simulink model "guidance_v1_4_1"  (R2019a)
settings: Solver=FixedStepDiscrete  StartTime=0.0  StopTime=inf  FixedStep=0.05  RelTol=1e-3  EnableMultiTasking=on
undefined symbols (not defined in the file or in its folder): Data, Data_SL_Info, Pose
libraries: robotlib x12, sharedtransform x1
settings Model: Creator=USER  LastModifiedBy=USER
settings DataIOCC: ReturnWorkspaceOutputs=off
settings OptimizationCC: EnhancedBackFolding=on  PassReuseOutputArgsAs=Individual arguments  MaxStackSize=64  OptimizeBlockOrder=speed  DifferentSizesBufferReuse=on  OptimizationCustomize=off
settings DebuggingCC: ParameterTunabilityLossMsg=error  PregeneratedLibrarySubsystemCodeDiagnostic=none  ArithmeticOperatorsInVariantConditions=warning
settings HardwareCC: ProdBitPerPointer=32  ProdBitPerSizeT=32  ProdBitPerPtrDiffT=32  ProdLargestAtomicFloat=None  ProdIntDivRoundTo=Undefined  ProdEndianess=Unspecified  ProdWordSize=32  ProdHWDeviceType=Generic->Unspecified (assume 32-bit Generic)
settings SFSimCC: SimUseLocalCustomCode=off  MATLABDynamicMemAlloc=off
settings RTWCC: SystemTargetFile=ert.tlc  HardwareBoard=Robot Operating System (ROS)  TLCOptions="-aInlineSetEventsForThisBaseRateFcn=TLC_FALSE -aSuppressMultiTaskScheduler=TLC_FALSE  -aRateBasedStepFcn=0"  TemplateMakefile=ert_default_tmf  GenerateReport=on  RTWUseLocalCustomCode=off  Toolchain=Catkin  BuildConfiguration=Faster Runs  IncludeHyperlinkInReport=on  LaunchReport=on  TargetLang=C++  GenerateTraceInfo=on  GenerateTraceReport=on  GenerateTraceReportSl=on  GenerateTraceReportSf=on  GenerateTraceReportEml=on
settings CodeAppCC: ForceParamTrailComments=on  IgnoreCustomStorageClasses=off  OperatorAnnotations=on  SimulinkDataObjDesc=on  SFDataObjDesc=on  InsertBlockDesc=on
settings ERTTargetCC: SupportVariableSizeSignals=on

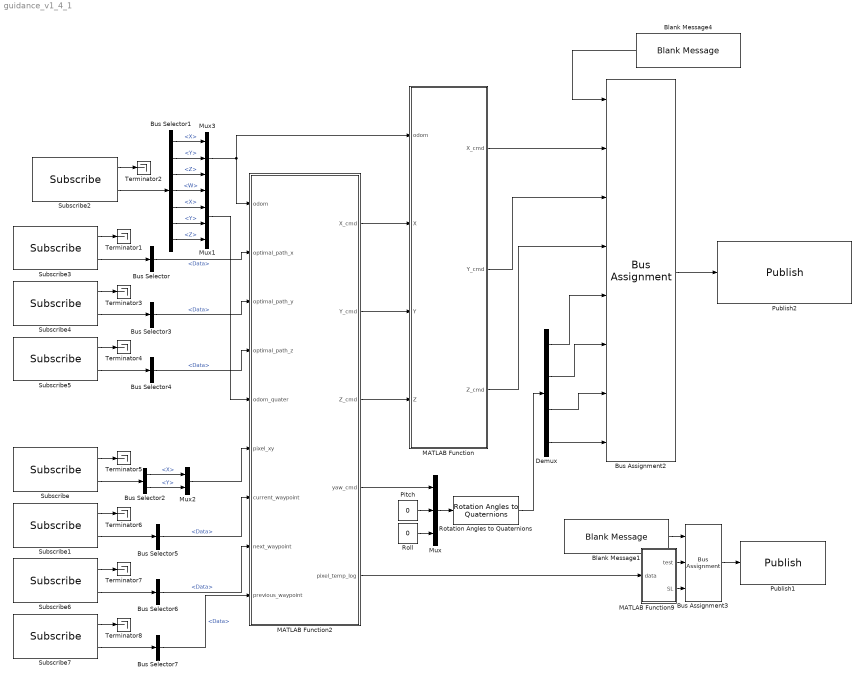
== system guidance_v1_4_1 ==
  " Roll" : Constant  Value=0  OutDataTypeStr=double  SampleTime=-1
  Blank Message1 : robotlib/Blank Message  messageClass=Message  entityType=std_msgs/Float32MultiArray  messageType=std_msgs/Float32MultiArray  SampleTime=-1
      settings: SourceProductBaseCode=RO
  Blank Message4 : robotlib/Blank Message  messageClass=Message  entityType=geometry_msgs/PoseStamped  messageType=geometry_msgs/PoseStamped  SampleTime=-1
      settings: SourceProductBaseCode=RO
  Bus Assignment2 : BusAssignment  AssignedSignals=Pose.Position.X,Pose.Position.Y,Pose.Position.Z,Pose.Orientation.W,Pose.Orientation.X,Pose.Orientation.Y,Pose.Orientation.Z
  Bus Assignment3 : BusAssignment  AssignedSignals=Data,Data_SL_Info.CurrentLength
  Bus Selector{,3..7} (6 alike) : BusSelector  OutputSignals=Data
  Bus Selector1 : BusSelector  OutputSignals=Pose.Pose.Position.X,Pose.Pose.Position.Y,Pose.Pose.Position.Z,Pose.Pose.Orientation.W,Pose.Pose.Orientation.X,Pose.Pose.Orientation.Y,Pose.Pose.Orientation.Z
  Bus Selector2 : BusSelector  OutputSignals=Pose.Position.X,Pose.Position.Y
  Demux : Demux
  MATLAB Function : MATLAB Function  TreatAsAtomicUnit=on
  MATLAB Function2 : MATLAB Function  TreatAsAtomicUnit=on
  MATLAB Function9 : MATLAB Function  TreatAsAtomicUnit=on
  Mux : Mux  Inputs=3
  Mux1 : Mux
  Mux2 : Mux  Inputs=2
  Mux3 : Mux  Inputs=3
  Pitch : Constant  Value=0  OutDataTypeStr=double  SampleTime=-1
  Publish1 : robotlib/Publish  topicSource=Specify your own  topic=/pixel_xy_log  messageType=std_msgs/Float32MultiArray  messageQueueLength=1
      settings: SourceProductBaseCode=RO
  Publish2 : robotlib/Publish  topicSource=Select from ROS network  topic=/mavros/setpoint_position/local  messageType=geometry_msgs/PoseStamped  messageQueueLength=1
      settings: SourceProductBaseCode=RO
  Rotation Angles to Quaternions : sharedtransform/Rotation Angles to Quaternions  rotationOrder=ZYX  aMode=aMode
      settings: SourceProductName=Aerospace Blockset  SourceProductBaseCode=AE
  Subscribe : robotlib/Subscribe  topicSource=Select from ROS network  topic=/pixel_XY  messageType=geometry_msgs/PoseStamped  sampleTime=-1  messageQueueLength=1
      settings: SourceProductBaseCode=RO
  Subscribe1 : robotlib/Subscribe  topicSource=Select from ROS network  topic=/current_point_cmd  messageType=std_msgs/Float32MultiArray  sampleTime=-1  messageQueueLength=1
      settings: SourceProductBaseCode=RO
  Subscribe2 : robotlib/Subscribe  topicSource=Select from ROS network  topic=/rtabmap/odom  messageType=nav_msgs/Odometry  sampleTime=-1  messageQueueLength=1
      settings: SourceProductBaseCode=RO
  Subscribe3 : robotlib/Subscribe  topicSource=Specify your own  topic=/optimal_path_x  messageType=std_msgs/Float32MultiArray  sampleTime=-1  messageQueueLength=1
      settings: SourceProductBaseCode=RO
  Subscribe4 : robotlib/Subscribe  topicSource=Specify your own  topic=/optimal_path_y  messageType=std_msgs/Float32MultiArray  sampleTime=-1  messageQueueLength=1
      settings: SourceProductBaseCode=RO
  Subscribe5 : robotlib/Subscribe  topicSource=Specify your own  topic=/optimal_path_z  messageType=std_msgs/Float32MultiArray  sampleTime=-1  messageQueueLength=1
      settings: SourceProductBaseCode=RO
  Subscribe6 : robotlib/Subscribe  topicSource=Select from ROS network  topic=/next_point_cmd  messageType=std_msgs/Float32MultiArray  sampleTime=-1  messageQueueLength=1
      settings: SourceProductBaseCode=RO
  Subscribe7 : robotlib/Subscribe  topicSource=Select from ROS network  topic=/previous_point_cmd  messageType=std_msgs/Float32MultiArray  sampleTime=-1  messageQueueLength=1
      settings: SourceProductBaseCode=RO
  Terminator{1..8} (8 alike) : Terminator
  wires:
  Subscribe2/1 -> Terminator2/1
  Subscribe2/2 -> Bus Selector1/1
  Subscribe3/2 -> Bus Selector/1
  Subscribe3/1 -> Terminator1/1
  Subscribe4/1 -> Terminator3/1
  Subscribe5/1 -> Terminator4/1
  Bus Assignment2/1 -> Publish2/1
  Subscribe4/2 -> Bus Selector3/1
  Subscribe5/2 -> Bus Selector4/1
  Bus Selector/1 -> MATLAB Function2/2(optimal_path_x)  "<Data>"
  Bus Selector3/1 -> MATLAB Function2/3(optimal_path_y)  "<Data>"
  Bus Selector4/1 -> MATLAB Function2/4(optimal_path_z)  "<Data>"
  Bus Selector1/1 -> Mux3/1  "<X>"
  Bus Selector1/2 -> Mux3/2  "<Y>"
  Bus Selector1/3 -> Mux3/3  "<Z>"
  Mux3/1 -> MATLAB Function2/1(odom), MATLAB Function/1(odom)
  Blank Message4/1 -> Bus Assignment2/1
  MATLAB Function2/4(yaw_cmd) -> Mux/1
  Mux/1 -> Rotation Angles to Quaternions/1
  Pitch/1 -> Mux/2
  " Roll"/1 -> Mux/3
  Rotation Angles to Quaternions/1 -> Demux/1
  Demux/1 -> Bus Assignment2/5
  Demux/2 -> Bus Assignment2/6
  Demux/3 -> Bus Assignment2/7
  Demux/4 -> Bus Assignment2/8
  Mux1/1 -> MATLAB Function2/5(odom_quater)
  Subscribe/1 -> Terminator5/1
  Subscribe/2 -> Bus Selector2/1
  Bus Selector2/1 -> Mux2/1  "<X>"
  Bus Selector2/2 -> Mux2/2  "<Y>"
  Mux2/1 -> MATLAB Function2/6(pixel_xy)
  Bus Selector1/4 -> Mux1/1  "<W>"
  Bus Selector1/5 -> Mux1/2  "<X>"
  Bus Selector1/6 -> Mux1/3  "<Y>"
  Bus Selector1/7 -> Mux1/4  "<Z>"
  MATLAB Function9/2(SL) -> Bus Assignment3/3
  MATLAB Function9/1(test) -> Bus Assignment3/2
  MATLAB Function2/5(pixel_temp_log) -> MATLAB Function9/1(data)
  Blank Message1/1 -> Bus Assignment3/1
  Bus Assignment3/1 -> Publish1/1
  MATLAB Function2/1(X_cmd) -> MATLAB Function/2(X)
  MATLAB Function2/2(Y_cmd) -> MATLAB Function/3(Y)
  MATLAB Function2/3(Z_cmd) -> MATLAB Function/4(Z)
  MATLAB Function/1(X_cmd) -> Bus Assignment2/2
  MATLAB Function/2(Y_cmd) -> Bus Assignment2/3
  MATLAB Function/3(Z_cmd) -> Bus Assignment2/4
  Subscribe1/1 -> Terminator6/1
  Subscribe6/1 -> Terminator7/1
  Subscribe1/2 -> Bus Selector5/1
  Subscribe6/2 -> Bus Selector6/1
  Bus Selector5/1 -> MATLAB Function2/7(current_waypoint)  "<Data>"
  Bus Selector6/1 -> MATLAB Function2/8(next_waypoint)  "<Data>"
  Subscribe7/1 -> Terminator8/1
  Bus Selector7/1 -> MATLAB Function2/9(previous_waypoint)  "<Data>"
  Subscribe7/2 -> Bus Selector7/1

== matlab function guidance_v1_4_1/MATLAB Function ==
  data: odom input; X_cmd output; X input; Y input; Z input; Y_cmd output; Z_cmd output
function [X_cmd,Y_cmd,Z_cmd] = fcn(odom,X,Y,Z)

persistent XYZ_temp
if isempty(XYZ_temp)
    XYZ_temp = [0,0,0];
end

% if isnan(XYZ_temp(1)) && sqrt(odom(1)^2+odom(2)^2) > 0.5 
if (XYZ_temp(3)<-0.5) 
%     X_cmd = nan;
%     Y_cmd = nan;
%     Z_cmd = nan;
    X_cmd = XYZ_temp(1);
    Y_cmd = XYZ_temp(2);
    Z_cmd = XYZ_temp(3);
else
    X_cmd = X;
    Y_cmd = Y;
    Z_cmd = Z;
end
XYZ_temp = [X_cmd,Y_cmd,Z_cmd];

== matlab function guidance_v1_4_1/MATLAB Function9 ==
  data: data input size=[10 1]; test output size=[1 128]; SL output
function [test,SL]   = func(data)

% test = single(nan(1,128));

test = single([data', nan(1,118)]);
% for i = 1:length(data)
%     test(i) = single(data(i));
% end

SL = uint32(length(data));


end

== matlab function guidance_v1_4_1/MATLAB Function2 ==
  data: X_cmd output; Y_cmd output; odom input; Z_cmd output; optimal_path_x input size=[128 1]; optimal_path_y input size=[128 1]; optimal_path_z input size=[128 1]; yaw_cmd output; odom_quater input; pixel_xy input; pixel_temp_log output; current_waypoint input; next_waypoint input; previous_waypoint input
function [X_cmd,Y_cmd,Z_cmd,yaw_cmd,pixel_temp_log] = fcn(odom,optimal_path_x,optimal_path_y,optimal_path_z,odom_quater,pixel_xy,current_waypoint,next_waypoint,previous_waypoint)

persistent yaw_mem yaw_inc hz_20 pixel_temp landing_hz

if isempty(yaw_mem)
    yaw_mem = 0;
    yaw_inc = 0;
    hz_20 = 0;
    pixel_temp = zeros(5,2);
    landing_hz = 0;
end

hz_20 = hz_20 + 1;
landing_hz = landing_hz +1;


% ----------------------------------------------------------------------
% Landing
% ----------------------------------------------------------------------
pixel_xy = pixel_xy';
if isempty(pixel_xy)
    pixel_xy = [0,0];
end
if landing_hz == 10
    landing_hz =0;
    pixel_temp = [pixel_xy; pixel_temp(1:4,:)];
end
euler_angle = quat2eul([odom_quater(1),odom_quater(2),odom_quater(3),odom_quater(4)]);

% if max(abs(pixel_temp),[],'all')<100 && (pixel_temp(1,1)~=pixel_temp(2,1) || pixel_temp(1,2) ~=pixel_temp(2,2)) && (pixel_temp(2,1)~=pixel_temp(3,1) || pixel_temp(2,2) ~=pixel_temp(3,2)) && (pixel_temp(3,1)~=pixel_temp(4,1) || pixel_temp(3,2) ~=pixel_temp(4,2)) && (pixel_temp(4,1)~=pixel_temp(5,1) || pixel_temp(4,2) ~=pixel_temp(5,2))
if max(abs(pixel_temp),[],'all')<80 && (pixel_temp(1,1)~=pixel_temp(2,1) || pixel_temp(1,2) ~=pixel_temp(2,2)) && (pixel_temp(2,1)~=pixel_temp(3,1) || pixel_temp(2,2) ~=pixel_temp(3,2)) && (pixel_temp(3,1)~=pixel_temp(4,1) || pixel_temp(3,2) ~=pixel_temp(4,2)) && (pixel_temp(4,1)~=pixel_temp(5,1) || pixel_temp(4,2) ~=pixel_temp(5,2))
%     Z_cmd = nan(1,1);
%     X_cmd = nan(1,1);
%     Y_cmd = nan(1,1);
    Z_cmd = -1;
    X_cmd = odom(1);
    Y_cmd = odom(2);
    yaw_cmd = euler_angle(1);
else
    if pixel_temp(1,1)~=pixel_temp(2,1) || pixel_temp(1,2) ~=pixel_temp(2,2)
        landing_x = odom(1)+(pixel_xy(2)*cos(euler_angle(1)) + -pixel_xy(1)*-sin(euler_angle(1)))*odom(3)/640;
        landing_y = odom(2)+(-pixel_xy(1)*cos(euler_angle(1)) + pixel_xy(2)*sin(euler_angle(1)))*odom(3)/640;
%         landing_x = odom(1)+(pixel_xy(2)*odom(3)/640 + 0.07)*cos(euler_angle(1)) + -pixel_xy(1)*odom(3)/640*-sin(euler_angle(1))  ;  % 카메라 오프셋 보정
%         landing_y = odom(2)+-pixel_xy(1)*odom(3)/640*cos(euler_angle(1)) + (pixel_xy(2)*odom(3)/640 + 0.07)*sin(euler_angle(1));
        Z_cmd = 1;
        X_cmd = landing_x;
        Y_cmd = landing_y;
        yaw_cmd = euler_angle(1);
    else
        % ----------------------------------------------------------------------
        % Traveling
        % ----------------------------------------------------------------------
        
        path_length = length(optimal_path_x);
        K = inf(path_length,1);
        optimal_path_norm = inf(path_length,3);
        
        % optimal_path_x_temp = optimal_path_x.Data';
        % optimal_path_y_temp = optimal_path_y.Data';
        
        optimal_path_norm(:,1) = single(optimal_path_x - odom(1));
        optimal_path_norm(:,2) = single(optimal_path_y - odom(2));
        optimal_path_norm(:,3) = single(optimal_path_z - odom(3));
        
        % optimal_path = [optimal_path_x' optimal_path_y'];
        % optimal_path_norm = optimal_path - [odom(1) odom(2)];
        
        for i=1:path_length
            K(i) = norm(optimal_path_norm(i,:));
        end
        
        [~,m] = min(K);
        
        % Z_cmd = optimal_path_z(m);
        if m >= 128
            m = 127;
        end
        
        % Z_cmd = double(optimal_path_z(m+1) + APF_vector(3));         % prediction
        % X_cmd = double(optimal_path_x(m+1) + APF_vector(1));
        % Y_cmd = double(optimal_path_y(m+1) + APF_vector(2));
        
        Z_cmd = double(optimal_path_z(m+1));         % prediction
        X_cmd = double(optimal_path_x(m+1));
        Y_cmd = double(optimal_path_y(m+1));
        
        if m <= 125
            %     yaw_vector1 = [optimal_path_x(m+1)-odom(1) optimal_path_y(m+1)-odom(2)] / norm([optimal_path_x(m+1)-odom(1) optimal_path_y(m+1)-odom(2)]);
            %     yaw_vector2 = [optimal_path_x(m+2)-odom(1) optimal_path_y(m+2)-odom(2)] / norm([optimal_path_x(m+2)-odom(1) optimal_path_y(m+2)-odom(2)]);
            %     yaw_vector3 = [optimal_path_x(m+3)-odom(1) optimal_path_y(m+3)-odom(2)] / norm([optimal_path_x(m+3)-odom(1) optimal_path_y(m+3)-odom(2)]);
            yaw_vector1 = [optimal_path_x(m+1)-odom(1) optimal_path_y(m+1)-odom(2)];
            yaw_vector2 = [optimal_path_x(m+2)-odom(1) optimal_path_y(m+2)-odom(2)];
            yaw_vector3 = [optimal_path_x(m+3)-odom(1) optimal_path_y(m+3)-odom(2)];
            yaw_vector = yaw_vector1 + yaw_vector2 + yaw_vector3;
            if norm(yaw_vector3) <= 0.4
                yaw_cmd = 0;
            else
                yaw_cmd = double( atan2(yaw_vector(2),yaw_vector(1)) );
            end
            yaw_mem = yaw_cmd;
            yaw_inc = 0;
            %     yaw_cmd = double( ( atan2(optimal_path_y(m+1)-odom(2),optimal_path_x(m+1)-odom(1)) + atan2(optimal_path_y(m+2)-odom(2),optimal_path_x(m+2)-odom(1)) + atan2(optimal_path_y(m+3)-odom(2),optimal_path_x(m+3)-odom(1)) ) / 3 );
        else
            yaw_cmd = yaw_mem + deg2rad(yaw_inc);
        end
        
        if hz_20 == 80
            hz_20 = 0;
            if m == 128
                yaw_inc = yaw_inc + 30;        % 4초마다 30도 돌려서 관찰
            end
        end
        
    end
end

% ----------------------------------------------------------------------
% Yaw command at changing waypoint
% ----------------------------------------------------------------------
if sqrt((odom(1)-current_waypoint(1))^2+(odom(2)-current_waypoint(2))^2)<0.8
%     yaw_cmd = double(atan2(next_waypoint(2)-odom(2),next_waypoint(1)-odom(1)));
    yaw_cmd = double(atan2(next_waypoint(2)-current_waypoint(2),next_waypoint(1)-current_waypoint(1)));
end
if sqrt((odom(1)-previous_waypoint(1))^2+(odom(2)-previous_waypoint(2))^2)<0.8
    yaw_cmd = double(atan2(current_waypoint(2)-previous_waypoint(2),current_waypoint(1)-previous_waypoint(1)));
end
% ----------------------------------------------------------------------
% Yaw saturation
% ----------------------------------------------------------------------
% yaw_difference = yaw_cmd - euler_angle(1);
% if yaw_difference > deg2rad(5)
%     yaw_cmd = euler_angle(1)+deg2rad(5);
% elseif yaw_difference < -deg2rad(5)
%     yaw_cmd = euler_angle(1)-deg2rad(5);
% end
% ----------------------------------------------------------------------
% Safety
% ----------------------------------------------------------------------

if odom(1) == 0 && odom(2) == 0 && odom(3) == 0
    Z_cmd = nan(1,1);
    X_cmd = nan(1,1);
    Y_cmd = nan(1,1);
end
pixel_temp_log = [pixel_temp(:,1);pixel_temp(:,2)];



end
